simulink model "functiondebug"  (R2024a)
settings: Solver=VariableStepAuto  StartTime=0.0  StopTime=10.0  RelTol=1e-3
libraries: simulink x1, mcbcontrolslib x1
settings Model: Creator=wsl  LastModifiedBy=wsl

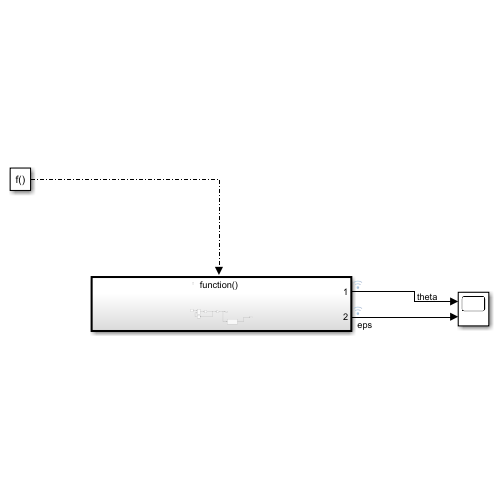
[thumbnail: Simulink's stored preview of the top-level diagram]
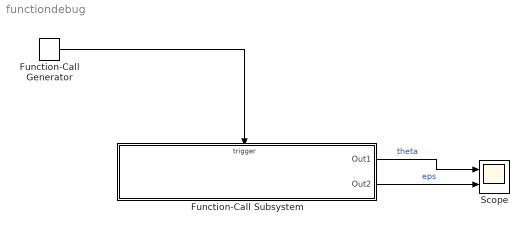
== system functiondebug ==
  Function-Call Generator : simulink/Ports & Subsystems/Function-Call Generator  sample_time=5e-5  numberOfIterations=1  DisallowWideOutput=off
  Function-Call Subsystem : Subsystem  TreatAsAtomicUnit=on
  Scope : Scope  NumInputPorts=2
  wires:
  Function-Call Generator/1 -> Function-Call Subsystem/Trigger
  Function-Call Subsystem/1(Out1) -> Scope/1  "theta"
  Function-Call Subsystem/2(Out2) -> Scope/2  "eps"

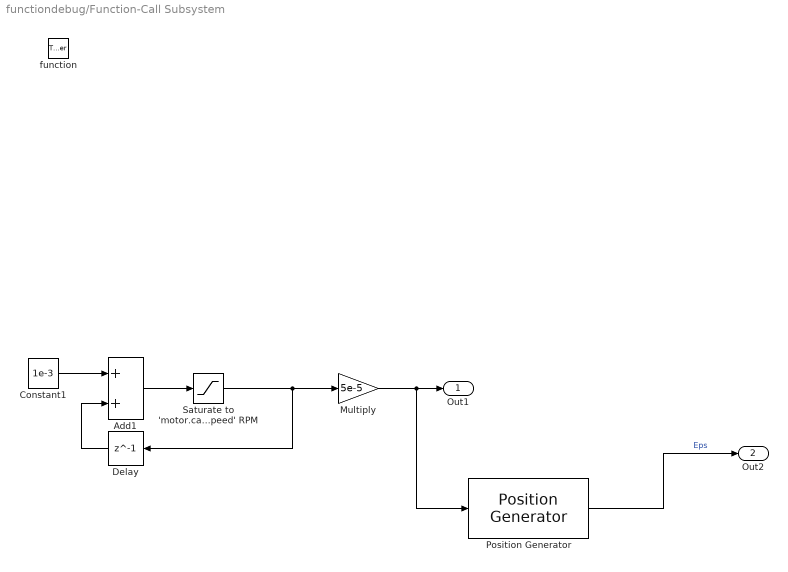
== system functiondebug/Function-Call Subsystem ==
  function : TriggerPort  TriggerType=function-call  VariantControl=(inherit)
  Add1 : Sum
  Constant1 : Constant  Value=1e-3  VectorParams1D=off  OutDataTypeStr=single
  Delay : Delay  DelayLength=1
  Multiply : Gain  Gain=5e-5  OutDataTypeStr=Inherit: Same as input
  Position Generator : mcbcontrolslib/Position Generator  AngleOutput=Per-unit  ExternalReset=none  Offset=0
  Saturate to 'motor.calibSpeed' RPM : Saturate  UpperLimit=2 *180/ 60  LowerLimit=0
  Out1 : Outport
  Out2 : Outport  Port=2
  wires:
  Multiply/1 -> Position Generator/1, Out1/1
  Add1/1 -> Saturate to 'motor.calibSpeed' RPM/1
  Delay/1 -> Add1/2
  Constant1/1 -> Add1/1
  Saturate to 'motor.calibSpeed' RPM/1 -> Delay/1, Multiply/1
  Position Generator/1 -> Out2/1  "Eps"
